simulink model "Subsystem"  (R2020b)
settings: Solver=FixedStepAuto  StartTime=0  StopTime=10  FixedStep=0.2  MaxStep=1  RelTol=1e-3
settings Model: Creator=Sudhanshu  LastModifiedBy=Sudhanshu
settings DataIOCC: SaveOutput=off  SaveTime=off

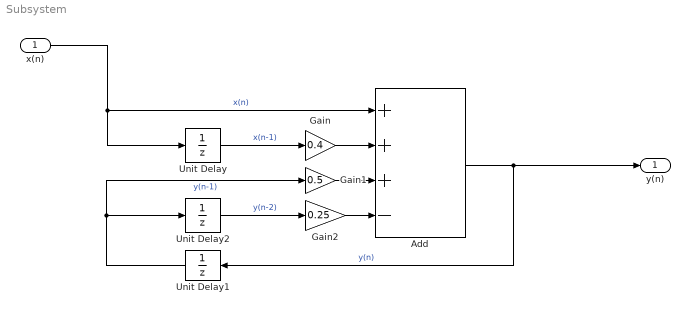
== system Subsystem ==
  x(n) : Inport  OutDataTypeStr=double  PortDimensions=1
  Add : Sum  Inputs=+++-
  Gain : Gain  Gain=0.4
  Gain1 : Gain  Gain=0.5
  Gain2 : Gain  Gain=0.25
  Unit Delay : UnitDelay  SampleTime=-1  HasFrameUpgradeWarning=on
  Unit Delay1 : UnitDelay  SampleTime=-1  HasFrameUpgradeWarning=on
  Unit Delay2 : UnitDelay  SampleTime=-1  HasFrameUpgradeWarning=on
  y(n) : Outport  OutDataTypeStr=double  PortDimensions=1  SampleTime=[0.20000000000000001,0]
  wires:
  Unit Delay/1 -> Gain/1  "x(n-1)"
  x(n)/1 -> Add/1, Unit Delay/1  "x(n)"
  Add/1 -> Unit Delay1/1, y(n)/1  "y(n)"
  Unit Delay1/1 -> Unit Delay2/1, Gain1/1  "y(n-1)"
  Gain/1 -> Add/2
  Unit Delay2/1 -> Gain2/1  "y(n-2)"
  Gain1/1 -> Add/3
  Gain2/1 -> Add/4
